simulink model "planar_robot_ct_disturabnce_esti_simulation"  (R2014a)
settings: Solver=ode45  StartTime=0.0  StopTime=50  FixedStep=0.0005  MaxStep=0.001  RelTol=1e-3
values from neighbouring files (symbols this model uses):
  a1 = u_gen(15)    [classical_joint_planar_robot_simulink.m]    (also in ct_gravit_inertia_planar_robot_simulink.m = u_gen(13); ct_gravit_planar_robot_simulink.m = u_gen(13); ct_pid_planar_robot_simulink.m; ct_planar_robot_simulink.m = u_gen(13))
  a2 = u_gen(16)    [classical_joint_planar_robot_simulink.m]    (also in ct_gravit_inertia_planar_robot_simulink.m = u_gen(14); ct_gravit_planar_robot_simulink.m = u_gen(14); ct_pid_planar_robot_simulink.m; ct_planar_robot_simulink.m = u_gen(14))
  b1 = u_gen(17)    [classical_joint_planar_robot_simulink.m]    (also in ct_gravit_inertia_planar_robot_simulink.m = u_gen(15); ct_gravit_planar_robot_simulink.m = u_gen(15); ct_pid_planar_robot_simulink.m; ct_planar_robot_simulink.m = u_gen(15))
  b2 = u_gen(18)    [classical_joint_planar_robot_simulink.m]    (also in ct_gravit_inertia_planar_robot_simulink.m = u_gen(16); ct_gravit_planar_robot_simulink.m = u_gen(16); ct_pid_planar_robot_simulink.m; ct_planar_robot_simulink.m = u_gen(16))
  g = u_gen(19)    [classical_joint_planar_robot_simulink.m]    (also in ct_gravit_inertia_planar_robot_simulink.m = u_gen(17); ct_gravit_planar_robot_simulink.m = u_gen(17); ct_pid_planar_robot_simulink.m; ct_planar_robot_simulink.m = u_gen(17))
  kp1 = wn1^2    [planar_robot_2dof.m]
  kp2 = wn2^2    [planar_robot_2dof.m]
  kv1 = 10    [planar_robot_2dof.m]
  kv2 = 10    [planar_robot_2dof.m]
  l1 = 100    [planar_robot_2dof.m]
  l2 = 100    [planar_robot_2dof.m]
  m1 = u_gen(11)    [ac_controller_simulink.m]    (also in classical_joint_planar_robot_simulink.m = u_gen(13); ct_gravit_inertia_planar_robot_simulink.m; ct_gravit_planar_robot_simulink.m; ct_pid_planar_robot_simulink.m = u_gen(13))
  M11 = eval((subs(M(1,1), q2, 0) + subs(M(1,1), q2, pi)))/2    [planar_robot_2dof.m]
  m2 = u_gen(12)    [ac_controller_simulink.m]    (also in classical_joint_planar_robot_simulink.m = u_gen(14); ct_gravit_inertia_planar_robot_simulink.m; ct_gravit_planar_robot_simulink.m; ct_pid_planar_robot_simulink.m = u_gen(14))
  M22 = eval(M(2,2))    [planar_robot_2dof.m]
settings Model: ExtModeTrigDuration=5000  Creator=Patrick  LastModifiedBy=Patrick
settings SolverCC: PositivePriorityOrder=on
settings RTWCC: SystemTargetFile=quarc_win64.tlc  TemplateMakefile=quarc_default_tmf  Description=QUARC Win64 Target  ProcessScript=quarc_win64_make_rtw_hook
settings STFCustomTargetCC: CombineOutputUpdateFcns=on  GRTInterface=off
settings GRTTargetCC: ParMdlRefBuildCompliant=off  CompOptLevelCompliant=off  MatFileLogging=off  CPPClassGenCompliant=off  ExtMode=on  ExtModeMexFile=quarc_comm

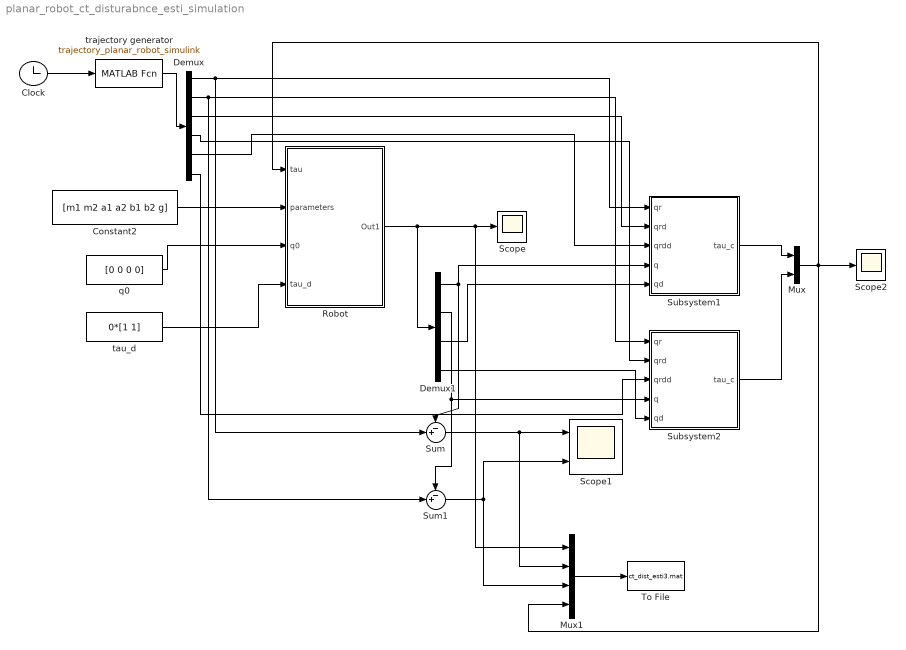
== system planar_robot_ct_disturabnce_esti_simulation ==
  Clock : Clock
  Constant2 : Constant  Value=[m1 m2 a1 a2 b1 b2 g]
  Demux : Demux  Outputs=6
  Demux1 : Demux
  Mux : Mux  Inputs=2
  Mux1 : Mux
  Robot : Subsystem
  Scope : Scope
      settings: YMin=-2.75  YMax=2.75
  Scope1 : Scope  NumInputPorts=2
      settings: TimeRange=10  YMin=-0.00025~-0.0002  YMax=0.00035~0.0002
  Scope2 : Scope
      settings: YMin=5  YMax=35  SaveName=ScopeData2
  Subsystem1 : Subsystem
  Subsystem2 : Subsystem
  Sum : Sum  Inputs=-+|
  Sum1 : Sum  Inputs=-+|
  To File : ToFile  Filename=ct_dist_esti3.mat  MatrixName=ct_de
  q0 : Constant  Value=[0 0 0 0]
  tau_d : Constant  Value=0*[1 1]
  trajectory generator : MATLABFcn  MATLABFcn=trajectory_planar_robot_simulink
  wires:
  Constant2/1 -> Robot/2(parameters)
  q0/1 -> Robot/3(q0)
  Robot/1(Out1) -> Demux1/1, Mux1/1, Scope/1
  Clock/1 -> trajectory generator/1
  trajectory generator/1 -> Demux/1
  Demux/1 -> Subsystem1/1(qr), Sum/2
  Sum/1 -> Mux1/2, Scope1/1
  Sum1/1 -> Scope1/2, Mux1/3
  Demux/2 -> Subsystem2/1(qr), Sum1/2
  tau_d/1 -> Robot/4(tau_d)
  Mux1/1 -> To File/1
  Demux1/1 -> Sum/1, Subsystem1/4(q)
  Demux1/2 -> Subsystem2/4(q), Sum1/1
  Demux/3 -> Subsystem1/2(qrd)
  Demux/5 -> Subsystem1/3(qrdd)
  Demux1/3 -> Subsystem1/5(qd)
  Subsystem1/1(tau_c) -> Mux/1
  Subsystem2/1(tau_c) -> Mux/2
  Mux/1 -> Scope2/1, Mux1/4, Robot/1(tau)
  Demux/4 -> Subsystem2/2(qrd)
  Demux/6 -> Subsystem2/3(qrdd)
  Demux1/4 -> Subsystem2/5(qd)

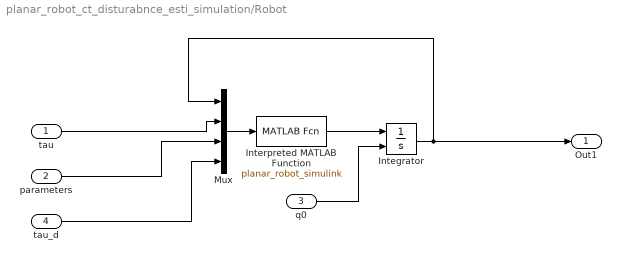
== system planar_robot_ct_disturabnce_esti_simulation/Robot ==
  tau : Inport
  parameters : Inport  Port=2
  q0 : Inport  Port=3
  tau_d : Inport  Port=4
  Integrator : Integrator  InitialConditionSource=external
  Interpreted MATLAB Function : MATLABFcn  MATLABFcn=planar_robot_simulink  OutputDimensions=4
  Mux : Mux
  Out1 : Outport
  wires:
  Interpreted MATLAB Function/1 -> Integrator/1
  tau/1 -> Mux/2
  q0/1 -> Integrator/2
  Mux/1 -> Interpreted MATLAB Function/1
  parameters/1 -> Mux/3
  Integrator/1 -> Out1/1, Mux/1
  tau_d/1 -> Mux/4

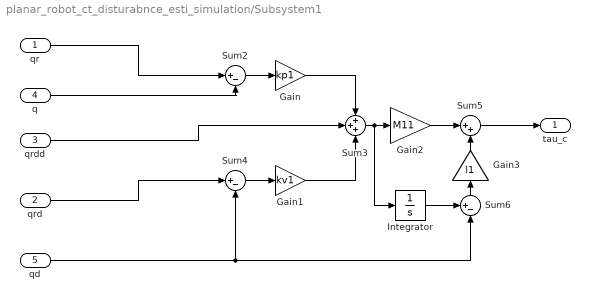
== system planar_robot_ct_disturabnce_esti_simulation/Subsystem1 ==
  qr : Inport
  qrd : Inport  Port=2
  qrdd : Inport  Port=3
  q : Inport  Port=4
  qd : Inport  Port=5
  Gain : Gain  Gain=kp1
  Gain1 : Gain  Gain=kv1
  Gain2 : Gain  Gain=M11
  Gain3 : Gain  Gain=l1
  Integrator : Integrator
  Sum2 : Sum  Inputs=|+-
  Sum3 : Sum  Inputs=+++
  Sum4 : Sum  Inputs=|+-
  Sum5 : Sum  Inputs=|++
  Sum6 : Sum  Inputs=+-|
  tau_c : Outport
  wires:
  Sum4/1 -> Gain1/1
  Sum3/1 -> Integrator/1, Gain2/1
  Gain2/1 -> Sum5/1
  Sum5/1 -> tau_c/1
  Gain/1 -> Sum3/1
  Sum2/1 -> Gain/1
  Gain3/1 -> Sum5/2
  q/1 -> Sum2/2
  Gain1/1 -> Sum3/3
  Integrator/1 -> Sum6/1
  qrdd/1 -> Sum3/2
  Sum6/1 -> Gain3/1
  qr/1 -> Sum2/1
  qrd/1 -> Sum4/1
  qd/1 -> Sum4/2, Sum6/2

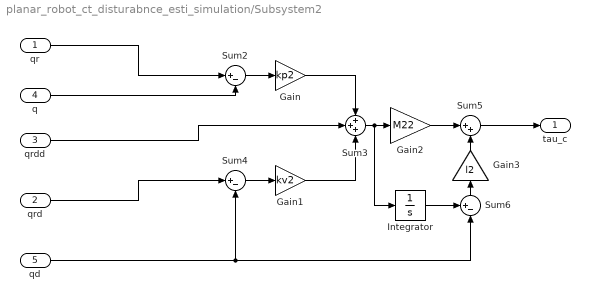
== system planar_robot_ct_disturabnce_esti_simulation/Subsystem2 ==
  qr : Inport
  qrd : Inport  Port=2
  qrdd : Inport  Port=3
  q : Inport  Port=4
  qd : Inport  Port=5
  Gain : Gain  Gain=kp2
  Gain1 : Gain  Gain=kv2
  Gain2 : Gain  Gain=M22
  Gain3 : Gain  Gain=l2
  Integrator : Integrator
  Sum2 : Sum  Inputs=|+-
  Sum3 : Sum  Inputs=+++
  Sum4 : Sum  Inputs=|+-
  Sum5 : Sum  Inputs=|++
  Sum6 : Sum  Inputs=+-|
  tau_c : Outport
  wires:
  Sum4/1 -> Gain1/1
  Sum3/1 -> Integrator/1, Gain2/1
  Gain2/1 -> Sum5/1
  Sum5/1 -> tau_c/1
  Gain/1 -> Sum3/1
  Sum2/1 -> Gain/1
  Gain3/1 -> Sum5/2
  q/1 -> Sum2/2
  Gain1/1 -> Sum3/3
  Integrator/1 -> Sum6/1
  qrdd/1 -> Sum3/2
  Sum6/1 -> Gain3/1
  qr/1 -> Sum2/1
  qrd/1 -> Sum4/1
  qd/1 -> Sum4/2, Sum6/2
